simulink model "SRSSwIndCtrl"  (R2018b)
settings: Solver=FixedStepDiscrete  StartTime=0.0  StopTime=10.0  FixedStep=0.01  RelTol=1e-3
undefined symbols (not defined in the file or in its folder): KeSMSuSRSMdSlctSwDurnTm_Val
settings Model: Creator=sn2xws  LastModifiedBy=sn2xws
settings Model: ModifiedHistory=|
  | CR269497
  | 23.4.13
  | 更改变量名：IfVeSMSeStPassCmprtMdRclRspStat为IfVeSMStPassCmprtMd_RfCtrl_Sw_RclRspStat
settings DataIOCC: SaveFormat=StructureWithTime
settings OptimizationCC: DefaultParameterBehavior=Inlined  EnhancedBackFolding=on  PassReuseOutputArgsAs=Individual arguments  ZeroExternalMemoryAtStartup=off  ZeroInternalMemoryAtStartup=off  OptimizeBlockOrder=speed  DifferentSizesBufferReuse=on  OptimizationCustomize=off
settings DebuggingCC: ParameterTunabilityLossMsg=error
settings HardwareCC: ProdBitPerPointer=32  ProdBitPerSizeT=32  ProdBitPerPtrDiffT=32  ProdLargestAtomicFloat=None  ProdWordSize=32  ProdHWDeviceType=Renesas->RH850
settings ModelReferenceCC: ModelReferenceNumInstancesAllowed=Single
settings SFSimCC: MATLABDynamicMemAlloc=off
settings RTWCC: SystemTargetFile=autosar.tlc  GenCodeOnly=on  TemplateMakefile=ert_default_tmf  Description=AUTOSAR  GenerateReport=on  IncludeHyperlinkInReport=on  LaunchReport=on  GenerateTraceInfo=on  GenerateTraceReport=on  GenerateTraceReportSl=on  GenerateTraceReportSf=on  GenerateTraceReportEml=on  GenerateCodeMetricsReport=on
settings CodeAppCC: ForceParamTrailComments=on  IgnoreCustomStorageClasses=off  OperatorAnnotations=on  SimulinkDataObjDesc=on  SFDataObjDesc=on  InsertBlockDesc=on
settings STFCustomTargetCC: TargetLangStandard=C99 (ISO)  MultiwordLength=256  ParMdlRefBuildCompliant=on  CompOptLevelCompliant=on  IncludeMdlTerminateFcn=off  CombineOutputUpdateFcns=on  SuppressErrorStatus=on  ERTCustomFileBanners=on  SupportNonFinite=off  SupportComplex=off  SupportContinuousTime=off  SupportNonInlinedSFcns=off  RemoveResetFunc=on  MATLABClassNameForMDSCustomization=Simulink.SoftwareTarget.ERTCustomization  AutosarCompliant=on  UseToolchainInfoCompliant=on  LookupTableObjectStructAxisOrder=2,1,3,4,...  LUTObjectStructOrderEvenSpacing=Size,Table,Breakpoints  SystemTargetFile=autosar.tlc
settings ERTTargetCC: TargetLangStandard=C99 (ISO)  ConcurrentExecutionCompliant=off  IncludeMdlTerminateFcn=off  SuppressErrorStatus=on  SupportNonFinite=off  SupportComplex=off  ModelStepFunctionPrototypeControlCompliant=off  CPPClassGenCompliant=off  AutosarCompliant=on  LookupTableObjectStructAxisOrder=2,1,3,4,...  LUTObjectStructOrderEvenSpacing=Size,Table,Breakpoints  InlinedParameterPlacement=NonHierarchical  ERTCustomFileTemplate=example_file_process.tlc  ERTFilePackagingFormat=Compact

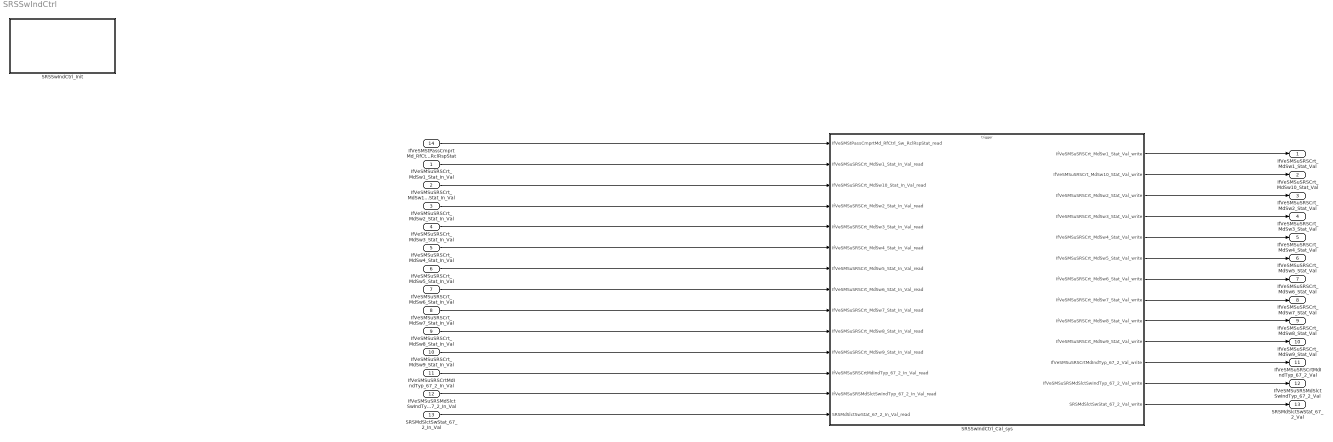
== system SRSSwIndCtrl ==
  IfVeSMSuSRSCrt_MdSw1_Stat_In_Val : Inport  OutDataTypeStr=uint8  PortDimensions=1
  IfVeSMSuSRSCrt_MdSw10_Stat_In_Val : Inport  Port=2  OutDataTypeStr=uint8  PortDimensions=1
  IfVeSMSuSRSCrt_MdSw2_Stat_In_Val : Inport  Port=3  OutDataTypeStr=uint8  PortDimensions=1
  IfVeSMSuSRSCrt_MdSw3_Stat_In_Val : Inport  Port=4  OutDataTypeStr=uint8  PortDimensions=1
  IfVeSMSuSRSCrt_MdSw4_Stat_In_Val : Inport  Port=5  OutDataTypeStr=uint8  PortDimensions=1
  IfVeSMSuSRSCrt_MdSw5_Stat_In_Val : Inport  Port=6  OutDataTypeStr=uint8  PortDimensions=1
  IfVeSMSuSRSCrt_MdSw6_Stat_In_Val : Inport  Port=7  OutDataTypeStr=uint8  PortDimensions=1
  IfVeSMSuSRSCrt_MdSw7_Stat_In_Val : Inport  Port=8  OutDataTypeStr=uint8  PortDimensions=1
  IfVeSMSuSRSCrt_MdSw8_Stat_In_Val : Inport  Port=9  OutDataTypeStr=uint8  PortDimensions=1
  IfVeSMSuSRSCrt_MdSw9_Stat_In_Val : Inport  Port=10  OutDataTypeStr=uint8  PortDimensions=1
  IfVeSMSuSRSCrtMdIndTyp_67_2_In_Val : Inport  Port=11  OutDataTypeStr=uint8  PortDimensions=1
  IfVeSMSuSRSMdSlctSwIndTyp_67_2_In_Val : Inport  Port=12  OutDataTypeStr=Enum: SRSSlctSwIndTyp  PortDimensions=1
  SRSMdSlctSwStat_67_2_In_Val : Inport  Port=13  OutDataTypeStr=Enum: SRSIndicatorStat  PortDimensions=1
  IfVeSMStPassCmprtMd_RfCtrl_Sw_RclRspStat : Inport  Port=14  OutDataTypeStr=uint8  PortDimensions=1
  SRSSwIndCtrl_Cal_sys : Subsystem
  SRSSwIndCtrl_Init : Subsystem
  IfVeSMSuSRSCrt_MdSw1_Stat_Val : Outport  OutDataTypeStr=uint8  PortDimensions=1
  IfVeSMSuSRSCrt_MdSw10_Stat_Val : Outport  Port=2  OutDataTypeStr=uint8  PortDimensions=1
  IfVeSMSuSRSCrt_MdSw2_Stat_Val : Outport  Port=3  OutDataTypeStr=uint8  PortDimensions=1
  IfVeSMSuSRSCrt_MdSw3_Stat_Val : Outport  Port=4  OutDataTypeStr=uint8  PortDimensions=1
  IfVeSMSuSRSCrt_MdSw4_Stat_Val : Outport  Port=5  OutDataTypeStr=uint8  PortDimensions=1
  IfVeSMSuSRSCrt_MdSw5_Stat_Val : Outport  Port=6  OutDataTypeStr=uint8  PortDimensions=1
  IfVeSMSuSRSCrt_MdSw6_Stat_Val : Outport  Port=7  OutDataTypeStr=uint8  PortDimensions=1
  IfVeSMSuSRSCrt_MdSw7_Stat_Val : Outport  Port=8  OutDataTypeStr=uint8  PortDimensions=1
  IfVeSMSuSRSCrt_MdSw8_Stat_Val : Outport  Port=9  OutDataTypeStr=uint8  PortDimensions=1
  IfVeSMSuSRSCrt_MdSw9_Stat_Val : Outport  Port=10  OutDataTypeStr=uint8  PortDimensions=1
  IfVeSMSuSRSCrtMdIndTyp_67_2_Val : Outport  Port=11  OutDataTypeStr=uint8  PortDimensions=1
  IfVeSMSuSRSMdSlctSwIndTyp_67_2_Val : Outport  Port=12  OutDataTypeStr=Enum: SRSSlctSwIndTyp  PortDimensions=1
  SRSMdSlctSwStat_67_2_Val : Outport  Port=13  OutDataTypeStr=Enum: SRSIndicatorStat  PortDimensions=1
  wires:
  IfVeSMSuSRSCrt_MdSw1_Stat_In_Val/1 -> SRSSwIndCtrl_Cal_sys/2(IfVeSMSuSRSCrt_MdSw1_Stat_In_Val_read)
  IfVeSMSuSRSCrt_MdSw10_Stat_In_Val/1 -> SRSSwIndCtrl_Cal_sys/3(IfVeSMSuSRSCrt_MdSw10_Stat_In_Val_read)
  IfVeSMSuSRSCrt_MdSw2_Stat_In_Val/1 -> SRSSwIndCtrl_Cal_sys/4(IfVeSMSuSRSCrt_MdSw2_Stat_In_Val_read)
  IfVeSMSuSRSCrt_MdSw3_Stat_In_Val/1 -> SRSSwIndCtrl_Cal_sys/5(IfVeSMSuSRSCrt_MdSw3_Stat_In_Val_read)
  IfVeSMSuSRSCrt_MdSw4_Stat_In_Val/1 -> SRSSwIndCtrl_Cal_sys/6(IfVeSMSuSRSCrt_MdSw4_Stat_In_Val_read)
  IfVeSMSuSRSCrt_MdSw5_Stat_In_Val/1 -> SRSSwIndCtrl_Cal_sys/7(IfVeSMSuSRSCrt_MdSw5_Stat_In_Val_read)
  IfVeSMSuSRSCrt_MdSw6_Stat_In_Val/1 -> SRSSwIndCtrl_Cal_sys/8(IfVeSMSuSRSCrt_MdSw6_Stat_In_Val_read)
  IfVeSMSuSRSCrt_MdSw7_Stat_In_Val/1 -> SRSSwIndCtrl_Cal_sys/9(IfVeSMSuSRSCrt_MdSw7_Stat_In_Val_read)
  IfVeSMSuSRSCrt_MdSw8_Stat_In_Val/1 -> SRSSwIndCtrl_Cal_sys/10(IfVeSMSuSRSCrt_MdSw8_Stat_In_Val_read)
  IfVeSMSuSRSCrt_MdSw9_Stat_In_Val/1 -> SRSSwIndCtrl_Cal_sys/11(IfVeSMSuSRSCrt_MdSw9_Stat_In_Val_read)
  IfVeSMSuSRSCrtMdIndTyp_67_2_In_Val/1 -> SRSSwIndCtrl_Cal_sys/12(IfVeSMSuSRSCrtMdIndTyp_67_2_In_Val_read)
  IfVeSMSuSRSMdSlctSwIndTyp_67_2_In_Val/1 -> SRSSwIndCtrl_Cal_sys/13(IfVeSMSuSRSMdSlctSwIndTyp_67_2_In_Val_read)
  SRSMdSlctSwStat_67_2_In_Val/1 -> SRSSwIndCtrl_Cal_sys/14(SRSMdSlctSwStat_67_2_In_Val_read)
  IfVeSMStPassCmprtMd_RfCtrl_Sw_RclRspStat/1 -> SRSSwIndCtrl_Cal_sys/1(IfVeSMStPassCmprtMd_RfCtrl_Sw_RclRspStat_read)
  SRSSwIndCtrl_Cal_sys/1(IfVeSMSuSRSCrt_MdSw1_Stat_Val_write) -> IfVeSMSuSRSCrt_MdSw1_Stat_Val/1
  SRSSwIndCtrl_Cal_sys/2(IfVeSMSuSRSCrt_MdSw10_Stat_Val_write) -> IfVeSMSuSRSCrt_MdSw10_Stat_Val/1
  SRSSwIndCtrl_Cal_sys/3(IfVeSMSuSRSCrt_MdSw2_Stat_Val_write) -> IfVeSMSuSRSCrt_MdSw2_Stat_Val/1
  SRSSwIndCtrl_Cal_sys/4(IfVeSMSuSRSCrt_MdSw3_Stat_Val_write) -> IfVeSMSuSRSCrt_MdSw3_Stat_Val/1
  SRSSwIndCtrl_Cal_sys/5(IfVeSMSuSRSCrt_MdSw4_Stat_Val_write) -> IfVeSMSuSRSCrt_MdSw4_Stat_Val/1
  SRSSwIndCtrl_Cal_sys/6(IfVeSMSuSRSCrt_MdSw5_Stat_Val_write) -> IfVeSMSuSRSCrt_MdSw5_Stat_Val/1
  SRSSwIndCtrl_Cal_sys/7(IfVeSMSuSRSCrt_MdSw6_Stat_Val_write) -> IfVeSMSuSRSCrt_MdSw6_Stat_Val/1
  SRSSwIndCtrl_Cal_sys/8(IfVeSMSuSRSCrt_MdSw7_Stat_Val_write) -> IfVeSMSuSRSCrt_MdSw7_Stat_Val/1
  SRSSwIndCtrl_Cal_sys/9(IfVeSMSuSRSCrt_MdSw8_Stat_Val_write) -> IfVeSMSuSRSCrt_MdSw8_Stat_Val/1
  SRSSwIndCtrl_Cal_sys/10(IfVeSMSuSRSCrt_MdSw9_Stat_Val_write) -> IfVeSMSuSRSCrt_MdSw9_Stat_Val/1
  SRSSwIndCtrl_Cal_sys/11(IfVeSMSuSRSCrtMdIndTyp_67_2_Val_write) -> IfVeSMSuSRSCrtMdIndTyp_67_2_Val/1
  SRSSwIndCtrl_Cal_sys/12(IfVeSMSuSRSMdSlctSwIndTyp_67_2_Val_write) -> IfVeSMSuSRSMdSlctSwIndTyp_67_2_Val/1
  SRSSwIndCtrl_Cal_sys/13(SRSMdSlctSwStat_67_2_Val_write) -> SRSMdSlctSwStat_67_2_Val/1

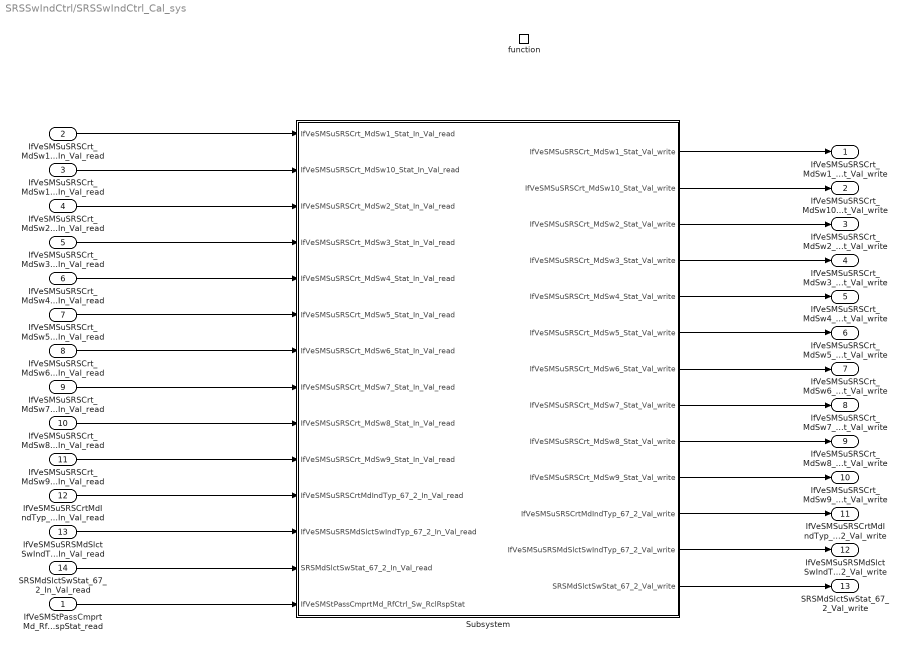
== system SRSSwIndCtrl/SRSSwIndCtrl_Cal_sys ==
  IfVeSMStPassCmprtMd_RfCtrl_Sw_RclRspStat_read : Inport
  IfVeSMSuSRSCrt_MdSw1_Stat_In_Val_read : Inport  Port=2
  IfVeSMSuSRSCrt_MdSw10_Stat_In_Val_read : Inport  Port=3
  IfVeSMSuSRSCrt_MdSw2_Stat_In_Val_read : Inport  Port=4
  IfVeSMSuSRSCrt_MdSw3_Stat_In_Val_read : Inport  Port=5
  IfVeSMSuSRSCrt_MdSw4_Stat_In_Val_read : Inport  Port=6
  IfVeSMSuSRSCrt_MdSw5_Stat_In_Val_read : Inport  Port=7
  IfVeSMSuSRSCrt_MdSw6_Stat_In_Val_read : Inport  Port=8
  IfVeSMSuSRSCrt_MdSw7_Stat_In_Val_read : Inport  Port=9
  IfVeSMSuSRSCrt_MdSw8_Stat_In_Val_read : Inport  Port=10
  IfVeSMSuSRSCrt_MdSw9_Stat_In_Val_read : Inport  Port=11
  IfVeSMSuSRSCrtMdIndTyp_67_2_In_Val_read : Inport  Port=12
  IfVeSMSuSRSMdSlctSwIndTyp_67_2_In_Val_read : Inport  Port=13
  SRSMdSlctSwStat_67_2_In_Val_read : Inport  Port=14
  function : TriggerPort  TriggerType=function-call  IsSimulinkFunction=on  FunctionName=SRSSwIndCtrl_Cal  VariantControl=(inherit)
  Subsystem : Subsystem
  IfVeSMSuSRSCrt_MdSw1_Stat_Val_write : Outport
      settings: EnsureOutportIsVirtual=on
  IfVeSMSuSRSCrt_MdSw10_Stat_Val_write : Outport  Port=2
      settings: EnsureOutportIsVirtual=on
  IfVeSMSuSRSCrt_MdSw2_Stat_Val_write : Outport  Port=3
      settings: EnsureOutportIsVirtual=on
  IfVeSMSuSRSCrt_MdSw3_Stat_Val_write : Outport  Port=4
      settings: EnsureOutportIsVirtual=on
  IfVeSMSuSRSCrt_MdSw4_Stat_Val_write : Outport  Port=5
      settings: EnsureOutportIsVirtual=on
  IfVeSMSuSRSCrt_MdSw5_Stat_Val_write : Outport  Port=6
      settings: EnsureOutportIsVirtual=on
  IfVeSMSuSRSCrt_MdSw6_Stat_Val_write : Outport  Port=7
      settings: EnsureOutportIsVirtual=on
  IfVeSMSuSRSCrt_MdSw7_Stat_Val_write : Outport  Port=8
      settings: EnsureOutportIsVirtual=on
  IfVeSMSuSRSCrt_MdSw8_Stat_Val_write : Outport  Port=9
      settings: EnsureOutportIsVirtual=on
  IfVeSMSuSRSCrt_MdSw9_Stat_Val_write : Outport  Port=10
      settings: EnsureOutportIsVirtual=on
  IfVeSMSuSRSCrtMdIndTyp_67_2_Val_write : Outport  Port=11
      settings: EnsureOutportIsVirtual=on
  IfVeSMSuSRSMdSlctSwIndTyp_67_2_Val_write : Outport  Port=12
      settings: EnsureOutportIsVirtual=on
  SRSMdSlctSwStat_67_2_Val_write : Outport  Port=13
      settings: EnsureOutportIsVirtual=on
  wires:
  SRSMdSlctSwStat_67_2_In_Val_read/1 -> Subsystem/13(SRSMdSlctSwStat_67_2_In_Val_read)
  IfVeSMSuSRSCrt_MdSw9_Stat_In_Val_read/1 -> Subsystem/10(IfVeSMSuSRSCrt_MdSw9_Stat_In_Val_read)
  IfVeSMSuSRSCrtMdIndTyp_67_2_In_Val_read/1 -> Subsystem/11(IfVeSMSuSRSCrtMdIndTyp_67_2_In_Val_read)
  IfVeSMSuSRSMdSlctSwIndTyp_67_2_In_Val_read/1 -> Subsystem/12(IfVeSMSuSRSMdSlctSwIndTyp_67_2_In_Val_read)
  IfVeSMSuSRSCrt_MdSw7_Stat_In_Val_read/1 -> Subsystem/8(IfVeSMSuSRSCrt_MdSw7_Stat_In_Val_read)
  IfVeSMSuSRSCrt_MdSw8_Stat_In_Val_read/1 -> Subsystem/9(IfVeSMSuSRSCrt_MdSw8_Stat_In_Val_read)
  IfVeSMSuSRSCrt_MdSw4_Stat_In_Val_read/1 -> Subsystem/5(IfVeSMSuSRSCrt_MdSw4_Stat_In_Val_read)
  IfVeSMSuSRSCrt_MdSw5_Stat_In_Val_read/1 -> Subsystem/6(IfVeSMSuSRSCrt_MdSw5_Stat_In_Val_read)
  IfVeSMSuSRSCrt_MdSw6_Stat_In_Val_read/1 -> Subsystem/7(IfVeSMSuSRSCrt_MdSw6_Stat_In_Val_read)
  IfVeSMSuSRSCrt_MdSw2_Stat_In_Val_read/1 -> Subsystem/3(IfVeSMSuSRSCrt_MdSw2_Stat_In_Val_read)
  IfVeSMSuSRSCrt_MdSw3_Stat_In_Val_read/1 -> Subsystem/4(IfVeSMSuSRSCrt_MdSw3_Stat_In_Val_read)
  IfVeSMStPassCmprtMd_RfCtrl_Sw_RclRspStat_read/1 -> Subsystem/14(IfVeSMStPassCmprtMd_RfCtrl_Sw_RclRspStat)
  IfVeSMSuSRSCrt_MdSw1_Stat_In_Val_read/1 -> Subsystem/1(IfVeSMSuSRSCrt_MdSw1_Stat_In_Val_read)
  IfVeSMSuSRSCrt_MdSw10_Stat_In_Val_read/1 -> Subsystem/2(IfVeSMSuSRSCrt_MdSw10_Stat_In_Val_read)
  Subsystem/1(IfVeSMSuSRSCrt_MdSw1_Stat_Val_write) -> IfVeSMSuSRSCrt_MdSw1_Stat_Val_write/1
  Subsystem/2(IfVeSMSuSRSCrt_MdSw10_Stat_Val_write) -> IfVeSMSuSRSCrt_MdSw10_Stat_Val_write/1
  Subsystem/3(IfVeSMSuSRSCrt_MdSw2_Stat_Val_write) -> IfVeSMSuSRSCrt_MdSw2_Stat_Val_write/1
  Subsystem/4(IfVeSMSuSRSCrt_MdSw3_Stat_Val_write) -> IfVeSMSuSRSCrt_MdSw3_Stat_Val_write/1
  Subsystem/5(IfVeSMSuSRSCrt_MdSw4_Stat_Val_write) -> IfVeSMSuSRSCrt_MdSw4_Stat_Val_write/1
  Subsystem/6(IfVeSMSuSRSCrt_MdSw5_Stat_Val_write) -> IfVeSMSuSRSCrt_MdSw5_Stat_Val_write/1
  Subsystem/7(IfVeSMSuSRSCrt_MdSw6_Stat_Val_write) -> IfVeSMSuSRSCrt_MdSw6_Stat_Val_write/1
  Subsystem/8(IfVeSMSuSRSCrt_MdSw7_Stat_Val_write) -> IfVeSMSuSRSCrt_MdSw7_Stat_Val_write/1
  Subsystem/9(IfVeSMSuSRSCrt_MdSw8_Stat_Val_write) -> IfVeSMSuSRSCrt_MdSw8_Stat_Val_write/1
  Subsystem/10(IfVeSMSuSRSCrt_MdSw9_Stat_Val_write) -> IfVeSMSuSRSCrt_MdSw9_Stat_Val_write/1
  Subsystem/11(IfVeSMSuSRSCrtMdIndTyp_67_2_Val_write) -> IfVeSMSuSRSCrtMdIndTyp_67_2_Val_write/1
  Subsystem/12(IfVeSMSuSRSMdSlctSwIndTyp_67_2_Val_write) -> IfVeSMSuSRSMdSlctSwIndTyp_67_2_Val_write/1
  Subsystem/13(SRSMdSlctSwStat_67_2_Val_write) -> SRSMdSlctSwStat_67_2_Val_write/1

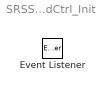
== system SRSSwIndCtrl/SRSSwIndCtrl_Init ==
  Event Listener : EventListener  EventName=reset

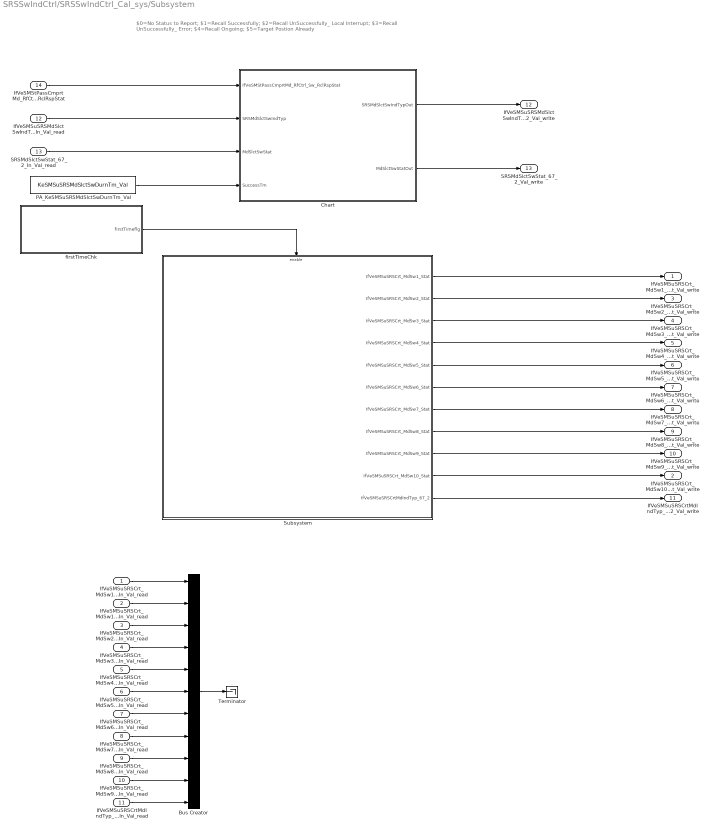
== system SRSSwIndCtrl/SRSSwIndCtrl_Cal_sys/Subsystem ==
  note: $0=No Status to Report; $1=Recall Successfully; $2=Recall UnSuccessfully_ Local Interrupt; $3=Recall UnSuccessfully_ Error; $4=Recall Ongoing; $5=Target Postion Already
  IfVeSMSuSRSCrt_MdSw1_Stat_In_Val_read : Inport
  IfVeSMSuSRSCrt_MdSw10_Stat_In_Val_read : Inport  Port=2
  IfVeSMSuSRSCrt_MdSw2_Stat_In_Val_read : Inport  Port=3
  IfVeSMSuSRSCrt_MdSw3_Stat_In_Val_read : Inport  Port=4
  IfVeSMSuSRSCrt_MdSw4_Stat_In_Val_read : Inport  Port=5
  IfVeSMSuSRSCrt_MdSw5_Stat_In_Val_read : Inport  Port=6
  IfVeSMSuSRSCrt_MdSw6_Stat_In_Val_read : Inport  Port=7
  IfVeSMSuSRSCrt_MdSw7_Stat_In_Val_read : Inport  Port=8
  IfVeSMSuSRSCrt_MdSw8_Stat_In_Val_read : Inport  Port=9
  IfVeSMSuSRSCrt_MdSw9_Stat_In_Val_read : Inport  Port=10
  IfVeSMSuSRSCrtMdIndTyp_67_2_In_Val_read : Inport  Port=11
  IfVeSMSuSRSMdSlctSwIndTyp_67_2_In_Val_read : Inport  Port=12
  SRSMdSlctSwStat_67_2_In_Val_read : Inport  Port=13
  IfVeSMStPassCmprtMd_RfCtrl_Sw_RclRspStat : Inport  Port=14
  Bus Creator : BusCreator  Inputs=11
  Chart : Stateflow chart  TreatAsAtomicUnit=on
  PA_KeSMSuSRSMdSlctSwDurnTm_Val : Constant  Value=KeSMSuSRSMdSlctSwDurnTm_Val
  Subsystem : Subsystem
  Terminator : Terminator
  firstTimeChk : Stateflow chart  TreatAsAtomicUnit=on
  IfVeSMSuSRSCrt_MdSw1_Stat_Val_write : Outport
      settings: EnsureOutportIsVirtual=on
  IfVeSMSuSRSCrt_MdSw10_Stat_Val_write : Outport  Port=2
      settings: EnsureOutportIsVirtual=on
  IfVeSMSuSRSCrt_MdSw2_Stat_Val_write : Outport  Port=3
      settings: EnsureOutportIsVirtual=on
  IfVeSMSuSRSCrt_MdSw3_Stat_Val_write : Outport  Port=4
      settings: EnsureOutportIsVirtual=on
  IfVeSMSuSRSCrt_MdSw4_Stat_Val_write : Outport  Port=5
      settings: EnsureOutportIsVirtual=on
  IfVeSMSuSRSCrt_MdSw5_Stat_Val_write : Outport  Port=6
      settings: EnsureOutportIsVirtual=on
  IfVeSMSuSRSCrt_MdSw6_Stat_Val_write : Outport  Port=7
      settings: EnsureOutportIsVirtual=on
  IfVeSMSuSRSCrt_MdSw7_Stat_Val_write : Outport  Port=8
      settings: EnsureOutportIsVirtual=on
  IfVeSMSuSRSCrt_MdSw8_Stat_Val_write : Outport  Port=9
      settings: EnsureOutportIsVirtual=on
  IfVeSMSuSRSCrt_MdSw9_Stat_Val_write : Outport  Port=10
      settings: EnsureOutportIsVirtual=on
  IfVeSMSuSRSCrtMdIndTyp_67_2_Val_write : Outport  Port=11
      settings: EnsureOutportIsVirtual=on
  IfVeSMSuSRSMdSlctSwIndTyp_67_2_Val_write : Outport  Port=12
      settings: EnsureOutportIsVirtual=on
  SRSMdSlctSwStat_67_2_Val_write : Outport  Port=13
      settings: EnsureOutportIsVirtual=on
  wires:
  IfVeSMSuSRSCrt_MdSw1_Stat_In_Val_read/1 -> Bus Creator/1
  IfVeSMSuSRSCrt_MdSw10_Stat_In_Val_read/1 -> Bus Creator/2
  IfVeSMSuSRSCrt_MdSw6_Stat_In_Val_read/1 -> Bus Creator/7
  IfVeSMSuSRSCrt_MdSw4_Stat_In_Val_read/1 -> Bus Creator/5
  IfVeSMSuSRSCrtMdIndTyp_67_2_In_Val_read/1 -> Bus Creator/11
  IfVeSMSuSRSCrt_MdSw5_Stat_In_Val_read/1 -> Bus Creator/6
  IfVeSMSuSRSCrt_MdSw8_Stat_In_Val_read/1 -> Bus Creator/9
  IfVeSMSuSRSCrt_MdSw2_Stat_In_Val_read/1 -> Bus Creator/3
  IfVeSMSuSRSCrt_MdSw7_Stat_In_Val_read/1 -> Bus Creator/8
  IfVeSMSuSRSCrt_MdSw9_Stat_In_Val_read/1 -> Bus Creator/10
  IfVeSMSuSRSCrt_MdSw3_Stat_In_Val_read/1 -> Bus Creator/4
  Chart/1(SRSMdSlctSwIndTypOut) -> IfVeSMSuSRSMdSlctSwIndTyp_67_2_Val_write/1
  Chart/2(MdSlctSwStatOut) -> SRSMdSlctSwStat_67_2_Val_write/1
  IfVeSMStPassCmprtMd_RfCtrl_Sw_RclRspStat/1 -> Chart/1(IfVeSMStPassCmprtMd_RfCtrl_Sw_RclRspStat)
  IfVeSMSuSRSMdSlctSwIndTyp_67_2_In_Val_read/1 -> Chart/2(SRSMdSlctSwIndTyp)
  SRSMdSlctSwStat_67_2_In_Val_read/1 -> Chart/3(MdSlctSwStat)
  PA_KeSMSuSRSMdSlctSwDurnTm_Val/1 -> Chart/4(SuccessTm)
  Bus Creator/1 -> Terminator/1
  Subsystem/1(IfVeSMSuSRSCrt_MdSw1_Stat) -> IfVeSMSuSRSCrt_MdSw1_Stat_Val_write/1
  Subsystem/11(IfVeSMSuSRSCrtMdIndTyp_67_2) -> IfVeSMSuSRSCrtMdIndTyp_67_2_Val_write/1
  Subsystem/2(IfVeSMSuSRSCrt_MdSw2_Stat) -> IfVeSMSuSRSCrt_MdSw2_Stat_Val_write/1
  Subsystem/3(IfVeSMSuSRSCrt_MdSw3_Stat) -> IfVeSMSuSRSCrt_MdSw3_Stat_Val_write/1
  Subsystem/4(IfVeSMSuSRSCrt_MdSw4_Stat) -> IfVeSMSuSRSCrt_MdSw4_Stat_Val_write/1
  Subsystem/5(IfVeSMSuSRSCrt_MdSw5_Stat) -> IfVeSMSuSRSCrt_MdSw5_Stat_Val_write/1
  Subsystem/6(IfVeSMSuSRSCrt_MdSw6_Stat) -> IfVeSMSuSRSCrt_MdSw6_Stat_Val_write/1
  Subsystem/7(IfVeSMSuSRSCrt_MdSw7_Stat) -> IfVeSMSuSRSCrt_MdSw7_Stat_Val_write/1
  Subsystem/8(IfVeSMSuSRSCrt_MdSw8_Stat) -> IfVeSMSuSRSCrt_MdSw8_Stat_Val_write/1
  Subsystem/9(IfVeSMSuSRSCrt_MdSw9_Stat) -> IfVeSMSuSRSCrt_MdSw9_Stat_Val_write/1
  Subsystem/10(IfVeSMSuSRSCrt_MdSw10_Stat) -> IfVeSMSuSRSCrt_MdSw10_Stat_Val_write/1
  firstTimeChk/1(firstTimeflg) -> Subsystem/Enable

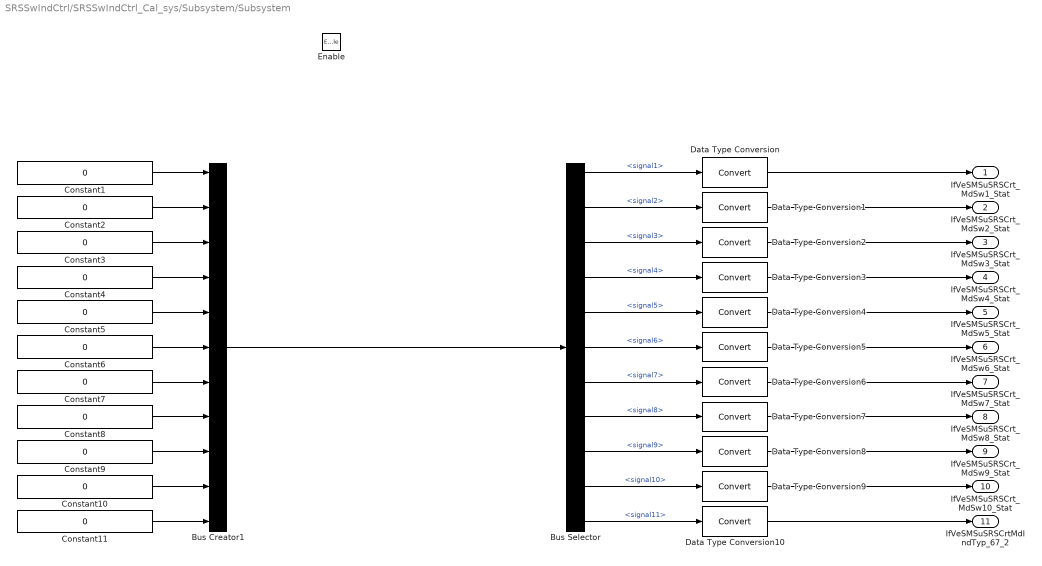
== system SRSSwIndCtrl/SRSSwIndCtrl_Cal_sys/Subsystem/Subsystem ==
  Enable : EnablePort
  Bus Creator1 : BusCreator  Inputs=11
  Bus Selector : BusSelector  OutputSignals=signal1,signal2,signal3,signal4,signal5,signal6,signal7,signal8,signal9,signal10,signal11
  Constant{1..11} (11 alike) : Constant  Value=0  OutDataTypeStr=uint8
  Data Type Conversion{,1..10} (11 alike) : DataTypeConversion
  IfVeSMSuSRSCrt_MdSw1_Stat : Outport
  IfVeSMSuSRSCrt_MdSw2_Stat : Outport  Port=2
  IfVeSMSuSRSCrt_MdSw3_Stat : Outport  Port=3
  IfVeSMSuSRSCrt_MdSw4_Stat : Outport  Port=4
  IfVeSMSuSRSCrt_MdSw5_Stat : Outport  Port=5
  IfVeSMSuSRSCrt_MdSw6_Stat : Outport  Port=6
  IfVeSMSuSRSCrt_MdSw7_Stat : Outport  Port=7
  IfVeSMSuSRSCrt_MdSw8_Stat : Outport  Port=8
  IfVeSMSuSRSCrt_MdSw9_Stat : Outport  Port=9
  IfVeSMSuSRSCrt_MdSw10_Stat : Outport  Port=10
  IfVeSMSuSRSCrtMdIndTyp_67_2 : Outport  Port=11
  wires:
  Bus Selector/1 -> Data Type Conversion/1  "<signal1>"
  Bus Creator1/1 -> Bus Selector/1
  Data Type Conversion7/1 -> IfVeSMSuSRSCrt_MdSw8_Stat/1
  Data Type Conversion/1 -> IfVeSMSuSRSCrt_MdSw1_Stat/1
  Constant6/1 -> Bus Creator1/6
  Bus Selector/8 -> Data Type Conversion7/1  "<signal8>"
  Constant5/1 -> Bus Creator1/5
  Bus Selector/11 -> Data Type Conversion10/1  "<signal11>"
  Constant1/1 -> Bus Creator1/1
  Bus Selector/5 -> Data Type Conversion4/1  "<signal5>"
  Constant2/1 -> Bus Creator1/2
  Constant4/1 -> Bus Creator1/4
  Constant11/1 -> Bus Creator1/11
  Constant10/1 -> Bus Creator1/10
  Data Type Conversion1/1 -> IfVeSMSuSRSCrt_MdSw2_Stat/1
  Data Type Conversion10/1 -> IfVeSMSuSRSCrtMdIndTyp_67_2/1
  Constant3/1 -> Bus Creator1/3
  Bus Selector/2 -> Data Type Conversion1/1  "<signal2>"
  Bus Selector/6 -> Data Type Conversion5/1  "<signal6>"
  Bus Selector/7 -> Data Type Conversion6/1  "<signal7>"
  Bus Selector/3 -> Data Type Conversion2/1  "<signal3>"
  Constant7/1 -> Bus Creator1/7
  Constant9/1 -> Bus Creator1/9
  Bus Selector/10 -> Data Type Conversion9/1  "<signal10>"
  Bus Selector/4 -> Data Type Conversion3/1  "<signal4>"
  Bus Selector/9 -> Data Type Conversion8/1  "<signal9>"
  Constant8/1 -> Bus Creator1/8
  Data Type Conversion2/1 -> IfVeSMSuSRSCrt_MdSw3_Stat/1
  Data Type Conversion6/1 -> IfVeSMSuSRSCrt_MdSw7_Stat/1
  Data Type Conversion3/1 -> IfVeSMSuSRSCrt_MdSw4_Stat/1
  Data Type Conversion5/1 -> IfVeSMSuSRSCrt_MdSw6_Stat/1
  Data Type Conversion8/1 -> IfVeSMSuSRSCrt_MdSw9_Stat/1
  Data Type Conversion4/1 -> IfVeSMSuSRSCrt_MdSw5_Stat/1
  Data Type Conversion9/1 -> IfVeSMSuSRSCrt_MdSw10_Stat/1

== stateflow chart SRSSwIndCtrl/SRSSwIndCtrl_Cal_sys/Subsystem/Chart ==
  note: IfVeSMStPassCmprtMd_RfCtrl_Sw_RclRspStat:$0=No Status to Report; $1=Recall Successfully; $2=Recall UnSuccessfully_ Local Interrupt; $3=Recall UnSuccessfully_ Error; $4=Recall Ongoing; $5=Target Postion Already
  state SwOut
    en:MdSlctSwStatOut=MdSlctSwStat;
    en:SRSMdSlctSwIndTypOut=SRSMdSlctSwIndTyp;
    du:MdSlctSwStatOut=MdSlctSwStat;
    du:SRSMdSlctSwIndTypOut=SRSMdSlctSwIndTyp;
  state MdStatOut
    state Success
      en:SRSMdSlctSwIndTypOut=SRSSlctSwIndTyp.Continuous;
  (default) -> SwOut : {TmpTmTick =SuccessTm*10;}
  SwOut -> Success [order 2] : [hasChangedTo(IfVeSMStPassCmprtMd_RfCtrl_Sw_RclRspStat,1)]
  SwOut -> Success [order 1] : [hasChangedTo(IfVeSMStPassCmprtMd_RfCtrl_Sw_RclRspStat,5)]
  Success -> SwOut : [after(TmpTmTick,tick)]
  MdStatOut -> SwOut : [hasChanged(MdSlctSwStat)&&MdSlctSwStat!=SRSIndicatorStat_NoIndicator]
  data: IfVeSMStPassCmprtMd_RfCtrl_Sw_RclRspStat input; SRSMdSlctSwIndTyp input; MdSlctSwStat input; SRSMdSlctSwIndTypOut output; MdSlctSwStatOut output; SuccessTm input; TmpTmTick local uint16

== stateflow chart SRSSwIndCtrl/SRSSwIndCtrl_Cal_sys/Subsystem/firstTimeChk ==
  (default) -> (junction 1)
  (junction 1) -> (junction 5) [order 1] : [chkflg ==0]
  (junction 1) -> (junction 3) [order 2] : {firstTimeflg = 0;}
  (junction 5) -> (junction 7) : {firstTimeflg = 1;
      | chkflg=1;}
  (junction 7) -> (junction 3)
  (junction 3) -> (junction 10)
  data: chkflg local boolean size=1; firstTimeflg output boolean size=1
